simulink model "Half_car_pitch"  (R2024b)
settings: Solver=VariableStepAuto  StartTime=0.0  StopTime=10  RelTol=1e-3
undefined symbols (not defined in the file): a, Af, b, Cf_sprung, Cl, Cr_sprung, I_PITCH, Kf_sprung, Kf_unsprung, Kr_sprung, Kr_unsprung, M_sprung, Mf_unsprung, Mr_unsprung, rho
settings Model: Creator=kanishka  LastModifiedBy=kanishka

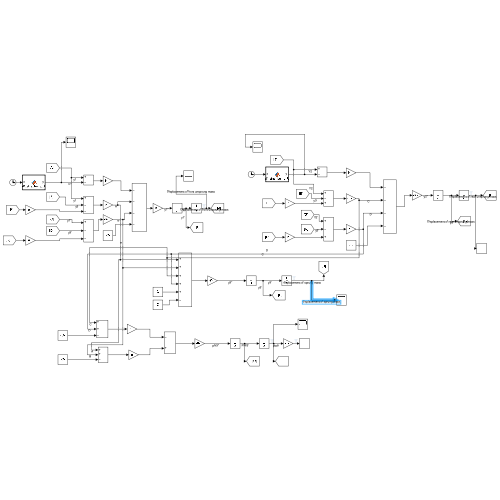
[thumbnail: Simulink's stored preview of the top-level diagram]
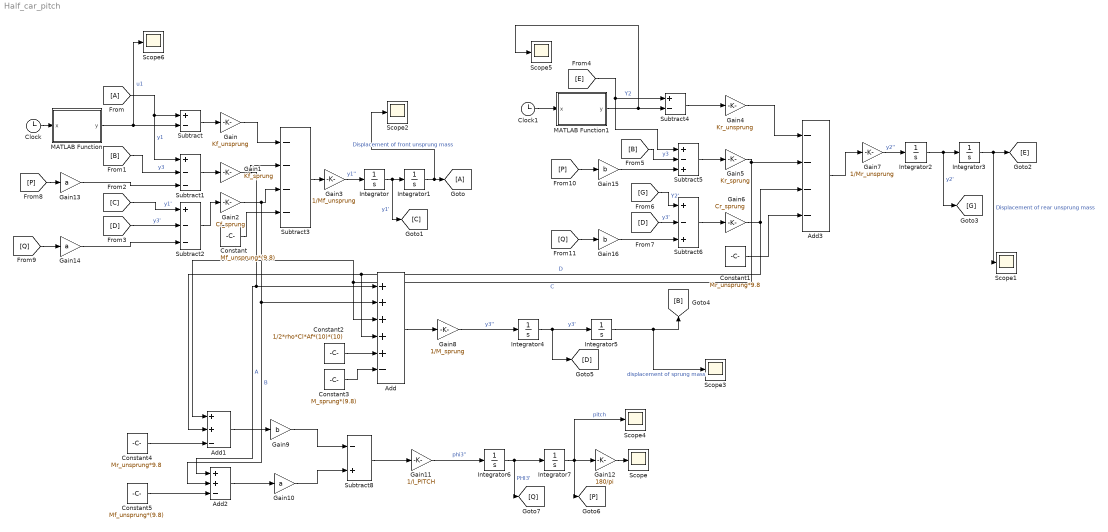
== system Half_car_pitch ==
  Add : Sum  Inputs=+++++-
  Add1 : Sum  Inputs=++-
  Add2 : Sum  Inputs=++-
  Add3 : Sum  Inputs=----
  Clock : Clock
  Clock1 : Clock
  Constant : Constant  Value=Mf_unsprung*(9.8)
  Constant1 : Constant  Value=Mr_unsprung*9.8
  Constant2 : Constant  Value=1/2*rho*Cl*Af*(10)*(10)
  Constant3 : Constant  Value=M_sprung*(9.8)
  Constant4 : Constant  Value=Mr_unsprung*9.8
  Constant5 : Constant  Value=Mf_unsprung*(9.8)
  From : From
  Gain : Gain  Gain=Kf_unsprung
  Gain1 : Gain  Gain=Kf_sprung
  Gain10 : Gain  Gain=a
  Gain11 : Gain  Gain=1/I_PITCH
  Gain12 : Gain  Gain=180/pi
  Gain13 : Gain  Gain=a
  Gain14 : Gain  Gain=a
  Gain15 : Gain  Gain=b
  Gain16 : Gain  Gain=b
  Gain2 : Gain  Gain=Cf_sprung
  Gain3 : Gain  Gain=1/Mf_unsprung
  Gain4 : Gain  Gain=Kr_unsprung
  Gain5 : Gain  Gain=Kr_sprung
  Gain6 : Gain  Gain=Cr_sprung
  Gain7 : Gain  Gain=1/Mr_unsprung
  Gain8 : Gain  Gain=1/M_sprung
  Gain9 : Gain  Gain=b
  Goto : Goto
  Integrator{,1..7} (8 alike) : Integrator
  MATLAB Function : MATLAB Function  TreatAsAtomicUnit=on
  MATLAB Function1 : MATLAB Function  TreatAsAtomicUnit=on
  Scope{,1..6} (7 alike) : Scope
  Subtract : Sum  Inputs=+-
  Subtract1 : Sum  Inputs=+--
  Subtract2 : Sum  Inputs=+--
  Subtract3 : Sum  Inputs=----
  Subtract4 : Sum  Inputs=+-
  Subtract5 : Sum  Inputs=+-+
  Subtract6 : Sum  Inputs=+-+
  Subtract8 : Sum  Inputs=-+
  wires:
  From/1 -> Subtract1/1, Subtract/1  "y1"
  MATLAB Function/1(y) -> Scope6/1, Subtract/2  "u1"
  Subtract/1 -> Gain/1
  [B] -> Subtract1/2  "y3"
  Subtract1/1 -> Gain1/1
  [C] -> Subtract2/1  "y1'"
  [D] -> Subtract2/2  "y3'"
  Subtract2/1 -> Gain2/1
  Gain/1 -> Subtract3/1
  Gain1/1 -> Subtract3/2, Add2/1, Add/1  "A"
  Gain2/1 -> Subtract3/3, Add/2, Add2/2  "B"
  Subtract3/1 -> Gain3/1
  Constant/1 -> Subtract3/4
  Gain3/1 -> Integrator/1  "y1''"
  Integrator/1 -> [C], Integrator1/1  "y1'"
  Integrator1/1 -> Scope2/1, Goto/1  "Displacement of front unsprung mass"
  [E] -> Subtract4/1, Subtract5/1  "Y2"
  MATLAB Function1/1(y) -> Scope5/1, Subtract4/2
  Subtract4/1 -> Gain4/1
  [B] -> Subtract5/2  "y3"
  Subtract5/1 -> Gain5/1
  [G] -> Subtract6/1  "Y2'"
  [D] -> Subtract6/2  "y3'"
  Gain4/1 -> Add3/1
  Gain5/1 -> Add3/2, Add1/1, Add/3  "C"
  Constant1/1 -> Add3/4
  Integrator2/1 -> Integrator3/1, [G]  "y2'"
  Gain7/1 -> Integrator2/1  "y2''"
  Integrator3/1 -> [E], Scope1/1  "Displacement of rear unsprung mass"
  Gain6/1 -> Add3/3, Add1/2, Add/4  "D"
  Constant2/1 -> Add/5
  Constant3/1 -> Add/6
  Add/1 -> Gain8/1
  Gain8/1 -> Integrator4/1  "y3''"
  Integrator4/1 -> [D], Integrator5/1  "y3'"
  Integrator5/1 -> Scope3/1, [B]  "displacement of sprung mass"
  Constant4/1 -> Add1/3
  Add1/1 -> Gain9/1
  Gain9/1 -> Subtract8/1
  Constant5/1 -> Add2/3
  Add2/1 -> Gain10/1
  Gain10/1 -> Subtract8/2
  Subtract8/1 -> Gain11/1
  Gain11/1 -> Integrator6/1  "phi3''"
  Integrator6/1 -> [Q], Integrator7/1  "PHI3'"
  Integrator7/1 -> Scope4/1, [P], Gain12/1  "pitch"
  Clock/1 -> MATLAB Function/1(x)
  Clock1/1 -> MATLAB Function1/1(x)
  Gain12/1 -> Scope/1
  Gain13/1 -> Subtract1/3
  [P] -> Gain13/1
  [Q] -> Gain14/1
  Gain14/1 -> Subtract2/3
  Subtract6/1 -> Gain6/1
  Add3/1 -> Gain7/1
  Gain15/1 -> Subtract5/3
  [P] -> Gain15/1
  Gain16/1 -> Subtract6/3
  [Q] -> Gain16/1

== matlab function Half_car_pitch/MATLAB Function ==
  data: x input; y output
function y = half_sine_bump_U1(x)

amplitude = 0.05;     
wavelength = 0.6;      
                




% Generate half sine wave profile for 0 <= x <= 0.3
if x >= 0 && x <= wavelength/2
    y = amplitude * sin((2*pi * x) / wavelength);
else
    y = 0;
end
end

== matlab function Half_car_pitch/MATLAB Function1 ==
  data: x input; y output
function y = half_sine_bump_U2(x)
amplitude = 0.05;     
wavelength = 0.6;      
v = 10;                
L = 1.53/2;             





if x >= L && x <=L+(wavelength/2)
    y = amplitude * sin(2*pi * (x-L) / wavelength);
else
    y = 0;
end
end
